simulink model "namestanje_parametara"  (R2018a)
settings: Solver=VariableStepAuto  StartTime=0.0  StopTime=10.0  RelTol=1e-3
values from neighbouring files (symbols this model uses):
  A = [ 0   1   0   0   0   0   0 ... (first row only)    [HPS.m]
  a21 = -4*k/(3*Mt)    (= -53333.3333333)    [HPS.m]
  a22 = -(Bp+b)/Mt    (= -13)    [HPS.m]
  a23 = Ap/Mt    (= 0.00065)    [HPS.m]
  a24 = 4*k/(3*Mt)    (= 53333.3333333)    [HPS.m]
  a25 = b/Mt    (= 10)    [HPS.m]
  a32 = -4*Be*Ap/Vt    (= -8450000000)    [HPS.m]
  a33 = -4*Be*(Ctp+Kc)/Vt    (= -2.6)    [HPS.m]
  a51 = 4*k/(3*m)    (= 26666.6666667)    [HPS.m]
  a52 = b/m    (= 5)    [HPS.m]
  a54 = -10*k/(3*m)    (= -66666.6666667)    [HPS.m]
  a55 = -(b+mu)/m    (= -5.001)    [HPS.m]
  a56 = 2*k/m    (= 40000)    [HPS.m]
  a74 = 4*k/m    (= 80000)    [HPS.m]
  a76 = -6*k/m    (= -120000)    [HPS.m]
  a77 = -2*mu/m    (= -0.002)    [HPS.m]
  Ap = D*D*pi/4    (= 0.00384845100065)    [HPS.m]
  B = [0;0;b31;0;0;0;0]    [HPS.m]
  b31 = 4*Be*Kq*Kt/(R*r*Kf*Vt)    (= 401440000)    [HPS.m]
  Bp = 30    [HPS.m]
  C = [0,0,0,1,0,0,0]    [HPS.m]
  DD = Kp*Td    (= 0.3675)    [HPS.m]
  I = Kp/Ti    (= 4800)    [HPS.m]
  Kp = 0.6*Kkr    (= 84)    [HPS.m]
  Mt = 10    [HPS.m]
libraries: simulink x2
settings Model: Creator=test4  LastModifiedBy=test4

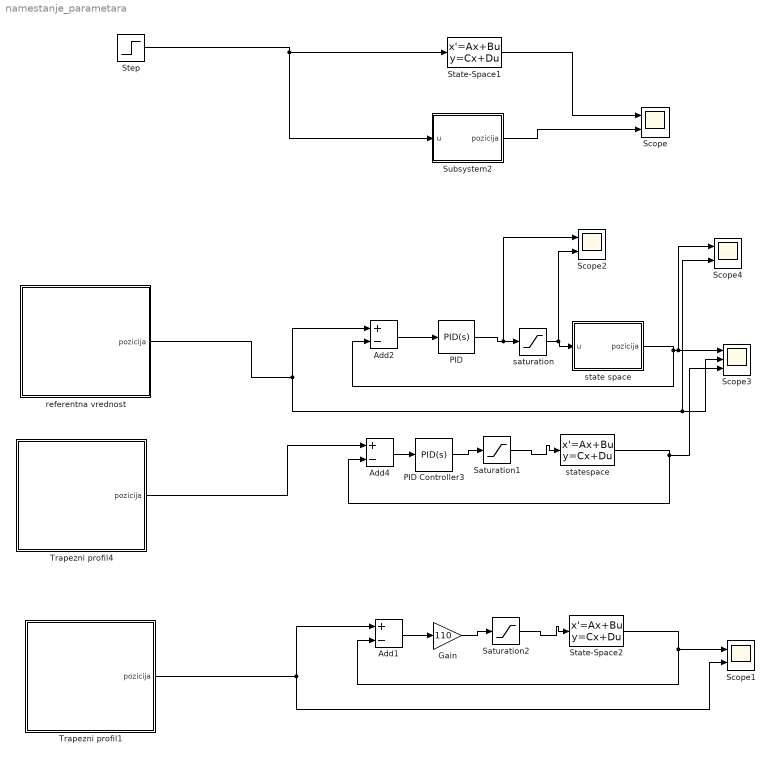
== system namestanje_parametara ==
  " PID" : simulink/Continuous/PID Controller  Controller=PID  TimeDomain=Continuous-time  SampleTime=-1  IntegratorMethod=Forward Euler  FilterMethod=Forward Euler  Form=Parallel  UseFilter=on  ControllerParametersSource=internal  P=Kp  I=I  D=DD  N=100  InitialConditionSource=internal  InitialConditionForIntegrator=0  InitialConditionForFilter=0  ExternalReset=none  LimitOutput=off  UpperSaturationLimit=inf  LowerSaturationLimit=-inf  LinearizeAsGain=on  AntiWindupMode=none  Kb=1  TrackingMode=off  Kt=1  PParamMin=[]  PParamMax=[]  IParamMin=[]  IParamMax=[]  DParamMin=[]  DParamMax=[]  NParamMin=[]  NParamMax=[]  KbParamMin=[]  KbParamMax=[]  KtParamMin=[]  KtParamMax=[]  POutMin=[]  POutMax=[]  IOutMin=[]  IOutMax=[]  DOutMin=[]  DOutMax=[]  NOutMin=[]  NOutMax=[]  KbOutMin=[]  KbOutMax=[]  KtOutMin=[]  KtOutMax=[]  IntegratorOutMin=[]  IntegratorOutMax=[]  FilterOutMin=[]  FilterOutMax=[]  SumOutMin=[]  SumOutMax=[]  SumI1OutMin=[]  SumI1OutMax=[]  SumI2OutMin=[]  SumI2OutMax=[]  SumI3OutMin=[]  SumI3OutMax=[]  SumDOutMin=[]  SumDOutMax=[]  SaturationOutMin=[]  SaturationOutMax=[]  IntegratorContinuousStateAttributes=''  IntegratorStateMustResolveToSignalObject=off  IntegratorRTWStateStorageClass=Auto  FilterContinuousStateAttributes=''  FilterStateMustResolveToSignalObject=off  FilterRTWStateStorageClass=Auto  DifferentiatorICPrevScaledInput=0  DifferentiatorOutMin=[]  DifferentiatorOutMax=[]  FilterDiffOutCoefMin=[]  FilterDiffOutCoefMax=[]  SumDenOutMin=[]  SumDenOutMax=[]  SumNumOutMin=[]  SumNumOutMax=[]  ReciprocalOutMin=[]  ReciprocalOutMax=[]  DivideOutMin=[]  DivideOutMax=[]  TunerSelectOption=Transfer Function Based (PID Tuner App)
  Add1 : Sum  Inputs=+-
  Add2 : Sum  Inputs=+-
  Add4 : Sum  Inputs=+-
  Gain : Gain  Gain=110
  PID Controller3 : simulink/Continuous/PID Controller  Controller=PID  TimeDomain=Continuous-time  SampleTime=-1  IntegratorMethod=Forward Euler  FilterMethod=Forward Euler  Form=Parallel  UseFilter=on  ControllerParametersSource=internal  P=Kp  I=I  D=DD  N=100  InitialConditionSource=internal  InitialConditionForIntegrator=0  InitialConditionForFilter=0  ExternalReset=none  LimitOutput=off  UpperSaturationLimit=inf  LowerSaturationLimit=-inf  LinearizeAsGain=on  AntiWindupMode=none  Kb=1  TrackingMode=off  Kt=1  PParamMin=[]  PParamMax=[]  IParamMin=[]  IParamMax=[]  DParamMin=[]  DParamMax=[]  NParamMin=[]  NParamMax=[]  KbParamMin=[]  KbParamMax=[]  KtParamMin=[]  KtParamMax=[]  POutMin=[]  POutMax=[]  IOutMin=[]  IOutMax=[]  DOutMin=[]  DOutMax=[]  NOutMin=[]  NOutMax=[]  KbOutMin=[]  KbOutMax=[]  KtOutMin=[]  KtOutMax=[]  IntegratorOutMin=[]  IntegratorOutMax=[]  FilterOutMin=[]  FilterOutMax=[]  SumOutMin=[]  SumOutMax=[]  SumI1OutMin=[]  SumI1OutMax=[]  SumI2OutMin=[]  SumI2OutMax=[]  SumI3OutMin=[]  SumI3OutMax=[]  SumDOutMin=[]  SumDOutMax=[]  SaturationOutMin=[]  SaturationOutMax=[]  IntegratorContinuousStateAttributes=''  IntegratorStateMustResolveToSignalObject=off  IntegratorRTWStateStorageClass=Auto  FilterContinuousStateAttributes=''  FilterStateMustResolveToSignalObject=off  FilterRTWStateStorageClass=Auto  DifferentiatorICPrevScaledInput=0  DifferentiatorOutMin=[]  DifferentiatorOutMax=[]  FilterDiffOutCoefMin=[]  FilterDiffOutCoefMax=[]  SumDenOutMin=[]  SumDenOutMax=[]  SumNumOutMin=[]  SumNumOutMax=[]  ReciprocalOutMin=[]  ReciprocalOutMax=[]  DivideOutMin=[]  DivideOutMax=[]  TunerSelectOption=Transfer Function Based (PID Tuner App)
  Saturation1 : Saturate  UpperLimit=24  LowerLimit=-24
  Saturation2 : Saturate  UpperLimit=24  LowerLimit=-24
  Scope{,1..2,4} (4 alike) : Scope  NumInputPorts=2
  Scope3 : Scope  NumInputPorts=3
  State-Space1 : StateSpace  A=A  B=B  C=C  D=0  InitialCondition=0
  State-Space2 : StateSpace  A=A  B=B  C=C  D=0  InitialCondition=0
  Step : Step  SampleTime=0
  Subsystem2 : Subsystem
  Trapezni profil1 : Subsystem
  Trapezni profil4 : Subsystem
  referentna vrednost : Subsystem
  saturation : Saturate  UpperLimit=24  LowerLimit=-24
  state space : Subsystem
  statespace : StateSpace  A=A  B=B  C=C  D=0  InitialCondition=0
  wires:
  State-Space1/1 -> Scope/1
  Subsystem2/1(pozicija) -> Scope/2
  Step/1 -> State-Space1/1, Subsystem2/1(u)
  " PID"/1 -> Scope2/1, saturation/1
  Trapezni profil1/1(pozicija) -> Scope1/2, Add1/1
  PID Controller3/1 -> Saturation1/1
  saturation/1 -> Scope2/2, state space/1(u)
  Gain/1 -> Saturation2/1
  Add2/1 -> " PID"/1
  Saturation1/1 -> statespace/1
  statespace/1 -> Scope3/3, Add4/2
  Add1/1 -> Gain/1
  Trapezni profil4/1(pozicija) -> Add4/1
  state space/1(pozicija) -> Scope4/1, Scope3/1, Add2/2
  referentna vrednost/1(pozicija) -> Add2/1, Scope4/2, Scope3/2
  Add4/1 -> PID Controller3/1
  State-Space2/1 -> Scope1/1, Add1/2
  Saturation2/1 -> State-Space2/1

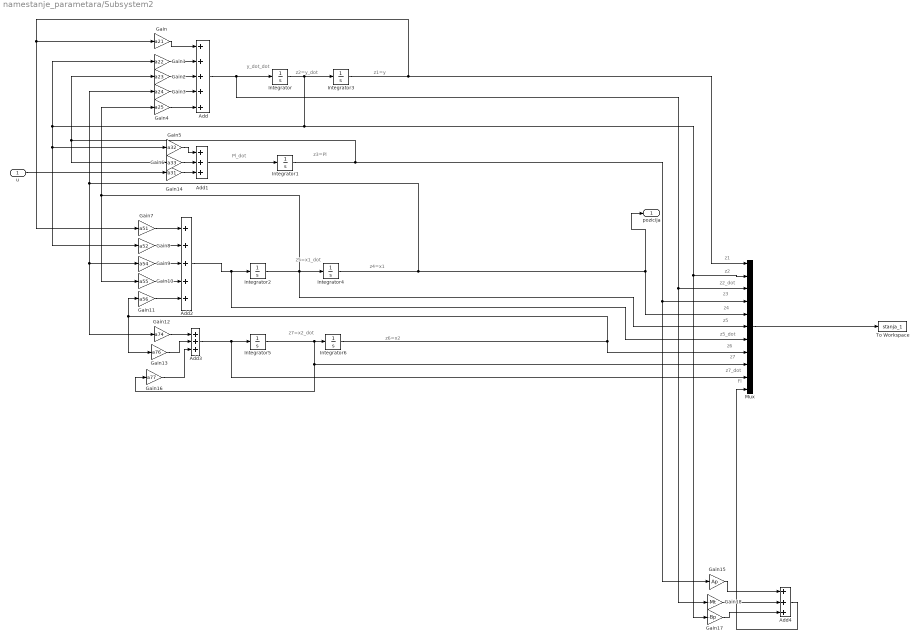
== system namestanje_parametara/Subsystem2 ==
  note: z3
  note: Fl
  note: z7_dot
  note: z7
  note: z6
  note: z5
  note: z4
  note: z2_dot
  note: z2
  note: z1
  note: z7=x2_dot
  note: z6=x2
  note: Pl_dot
  note: z5=x1_dot
  note: z4=x1
  note: y_dot_dot
  note: z3=Pl
  note: z1=y
  note: z2=y_dot
  note: z5_dot
  u : Inport
  Add : Sum  Inputs=+++++
  Add1 : Sum  Inputs=+++
  Add2 : Sum  Inputs=+++++
  Add3 : Sum  Inputs=+++
  Add4 : Sum  Inputs=+++
  Gain : Gain  Gain=a21
  Gain1 : Gain  Gain=a22
  Gain10 : Gain  Gain=a55
  Gain11 : Gain  Gain=a56
  Gain12 : Gain  Gain=a74
  Gain13 : Gain  Gain=a76
  Gain14 : Gain  Gain=b31
  Gain15 : Gain  Gain=Ap
  Gain16 : Gain  Gain=a77
  Gain17 : Gain  Gain=-Bp
  Gain18 : Gain  Gain=-Mt
  Gain2 : Gain  Gain=a23
  Gain3 : Gain  Gain=a24
  Gain4 : Gain  Gain=a25
  Gain5 : Gain  Gain=a32
  Gain6 : Gain  Gain=a33
  Gain7 : Gain  Gain=a51
  Gain8 : Gain  Gain=a52
  Gain9 : Gain  Gain=a54
  Integrator{,1..6} (7 alike) : Integrator
  Mux : Mux  Inputs=11
  To Workspace : ToWorkspace  VariableName=stanja_1  SampleTime=-1
  pozicija : Outport
  wires:
  Integrator/1 -> Mux/2, Gain17/1, Gain5/1, Gain8/1, Gain1/1, Integrator3/1
  Integrator4/1 -> Gain9/1, Gain12/1, Gain3/1, pozicija/1, Mux/5
  Gain13/1 -> Add3/2
  Gain4/1 -> Add/5
  Integrator5/1 -> Gain16/1, Mux/9, Integrator6/1
  Gain1/1 -> Add/2
  Add2/1 -> Mux/7, Integrator2/1
  Gain8/1 -> Add2/2
  Integrator6/1 -> Mux/8, Gain13/1, Gain11/1
  Add/1 -> Gain18/1, Mux/3, Integrator/1
  Gain6/1 -> Add1/2
  Gain2/1 -> Add/3
  Integrator1/1 -> Gain15/1, Mux/4, Gain6/1, Gain2/1
  Gain/1 -> Add/1
  Gain7/1 -> Add2/1
  Add3/1 -> Mux/10, Integrator5/1
  Gain10/1 -> Add2/4
  Add1/1 -> Integrator1/1
  Integrator3/1 -> Mux/1, Gain7/1, Gain/1
  Gain12/1 -> Add3/1
  Gain5/1 -> Add1/1
  Gain11/1 -> Add2/5
  Gain3/1 -> Add/4
  Gain9/1 -> Add2/3
  Integrator2/1 -> Mux/6, Integrator4/1, Gain4/1, Gain10/1
  Gain14/1 -> Add1/3
  u/1 -> Gain14/1
  Mux/1 -> To Workspace/1
  Gain18/1 -> Add4/2
  Gain15/1 -> Add4/1
  Gain17/1 -> Add4/3
  Add4/1 -> Mux/11
  Gain16/1 -> Add3/3

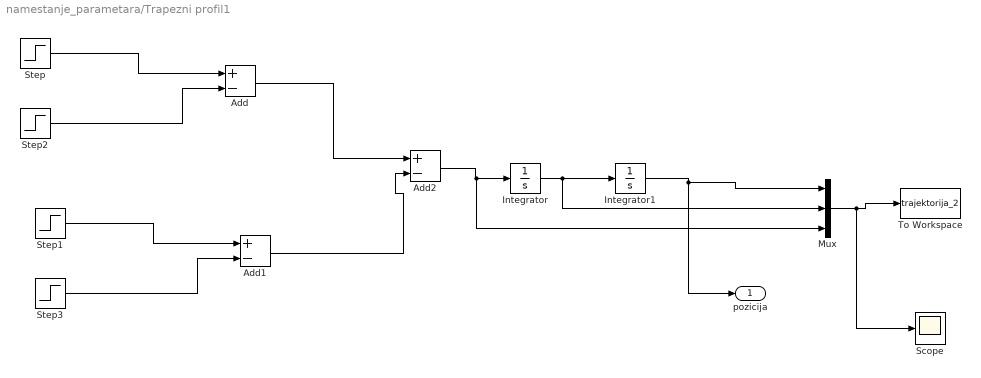
== system namestanje_parametara/Trapezni profil1 ==
  Add : Sum  Inputs=+-
  Add1 : Sum  Inputs=+-
  Add2 : Sum  Inputs=+-
  Integrator : Integrator
  Integrator1 : Integrator
  Mux : Mux  Inputs=3
  Scope : Scope
  Step : Step  Time=0  After=0.2667  SampleTime=0
  Step1 : Step  Time=1.5  After=0.2667  SampleTime=0
  Step2 : Step  Time=0.5  After=0.2667  SampleTime=0
  Step3 : Step  Time=2  After=0.2667  SampleTime=0
  To Workspace : ToWorkspace  VariableName=trajektorija_2  SampleTime=-1
  pozicija : Outport
  wires:
  Add1/1 -> Add2/2
  Step3/1 -> Add1/2
  Add/1 -> Add2/1
  Integrator1/1 -> Mux/1, pozicija/1
  Integrator/1 -> Mux/2, Integrator1/1
  Add2/1 -> Mux/3, Integrator/1
  Step1/1 -> Add1/1
  Step2/1 -> Add/2
  Step/1 -> Add/1
  Mux/1 -> Scope/1, To Workspace/1

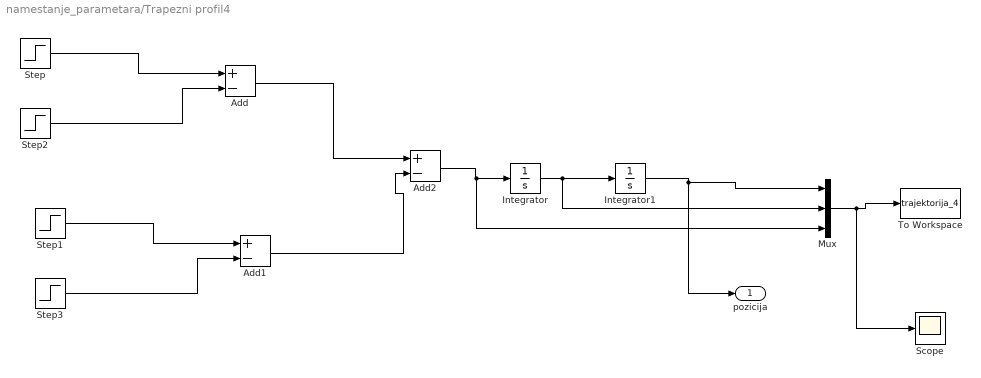
== system namestanje_parametara/Trapezni profil4 ==
  Add : Sum  Inputs=+-
  Add1 : Sum  Inputs=+-
  Add2 : Sum  Inputs=+-
  Integrator : Integrator
  Integrator1 : Integrator
  Mux : Mux  Inputs=3
  Scope : Scope
  Step : Step  Time=0  After=0.2667  SampleTime=0
  Step1 : Step  Time=1.5  After=0.2667  SampleTime=0
  Step2 : Step  Time=0.5  After=0.2667  SampleTime=0
  Step3 : Step  Time=2  After=0.2667  SampleTime=0
  To Workspace : ToWorkspace  VariableName=trajektorija_4  SampleTime=-1
  pozicija : Outport
  wires:
  Add1/1 -> Add2/2
  Step3/1 -> Add1/2
  Add/1 -> Add2/1
  Integrator1/1 -> Mux/1, pozicija/1
  Integrator/1 -> Mux/2, Integrator1/1
  Add2/1 -> Mux/3, Integrator/1
  Step1/1 -> Add1/1
  Step2/1 -> Add/2
  Step/1 -> Add/1
  Mux/1 -> Scope/1, To Workspace/1

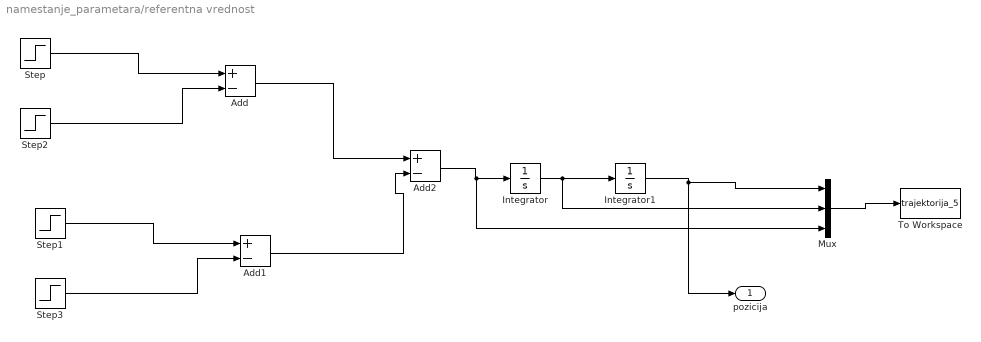
== system namestanje_parametara/referentna vrednost ==
  Add : Sum  Inputs=+-
  Add1 : Sum  Inputs=+-
  Add2 : Sum  Inputs=+-
  Integrator : Integrator
  Integrator1 : Integrator
  Mux : Mux  Inputs=3
  Step : Step  Time=0  After=0.2667  SampleTime=0
  Step1 : Step  Time=1.5  After=0.2667  SampleTime=0
  Step2 : Step  Time=0.5  After=0.2667  SampleTime=0
  Step3 : Step  Time=2  After=0.2667  SampleTime=0
  To Workspace : ToWorkspace  VariableName=trajektorija_5  SampleTime=-1
  pozicija : Outport
  wires:
  Add1/1 -> Add2/2
  Step3/1 -> Add1/2
  Add/1 -> Add2/1
  Integrator1/1 -> Mux/1, pozicija/1
  Integrator/1 -> Mux/2, Integrator1/1
  Add2/1 -> Mux/3, Integrator/1
  Step1/1 -> Add1/1
  Step2/1 -> Add/2
  Step/1 -> Add/1
  Mux/1 -> To Workspace/1

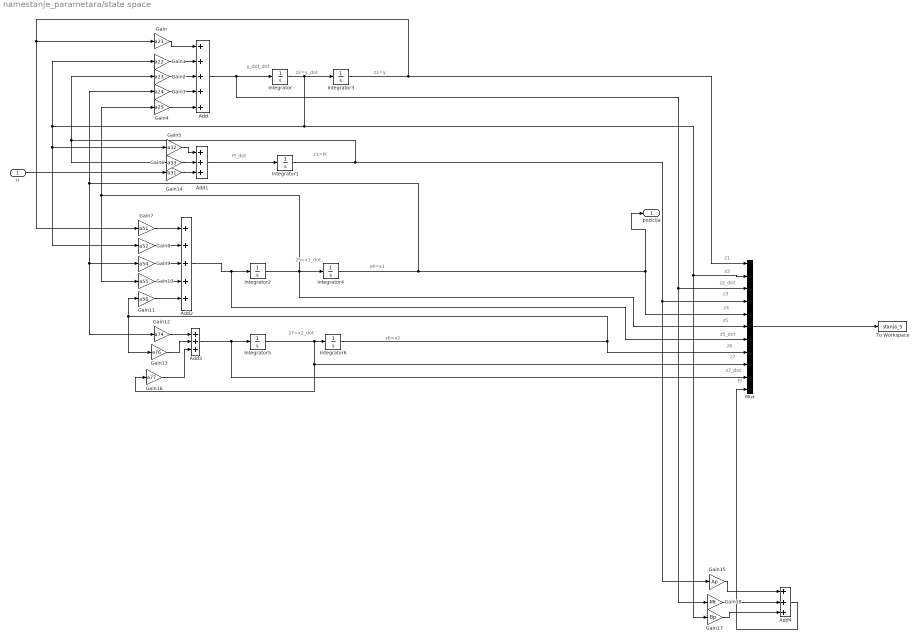
== system namestanje_parametara/state space ==
  note: z3
  note: Fl
  note: z7_dot
  note: z7
  note: z6
  note: z5
  note: z4
  note: z2_dot
  note: z2
  note: z1
  note: z7=x2_dot
  note: z6=x2
  note: Pl_dot
  note: z5=x1_dot
  note: z4=x1
  note: y_dot_dot
  note: z3=Pl
  note: z1=y
  note: z2=y_dot
  note: z5_dot
  u : Inport
  Add : Sum  Inputs=+++++
  Add1 : Sum  Inputs=+++
  Add2 : Sum  Inputs=+++++
  Add3 : Sum  Inputs=+++
  Add4 : Sum  Inputs=+++
  Gain : Gain  Gain=a21
  Gain1 : Gain  Gain=a22
  Gain10 : Gain  Gain=a55
  Gain11 : Gain  Gain=a56
  Gain12 : Gain  Gain=a74
  Gain13 : Gain  Gain=a76
  Gain14 : Gain  Gain=b31
  Gain15 : Gain  Gain=Ap
  Gain16 : Gain  Gain=a77
  Gain17 : Gain  Gain=-Bp
  Gain18 : Gain  Gain=-Mt
  Gain2 : Gain  Gain=a23
  Gain3 : Gain  Gain=a24
  Gain4 : Gain  Gain=a25
  Gain5 : Gain  Gain=a32
  Gain6 : Gain  Gain=a33
  Gain7 : Gain  Gain=a51
  Gain8 : Gain  Gain=a52
  Gain9 : Gain  Gain=a54
  Integrator{,1..6} (7 alike) : Integrator
  Mux : Mux  Inputs=11
  To Workspace : ToWorkspace  VariableName=stanja_5  SampleTime=-1
  pozicija : Outport
  wires:
  Integrator/1 -> Mux/2, Gain17/1, Gain5/1, Gain8/1, Gain1/1, Integrator3/1
  Integrator4/1 -> Gain9/1, Gain12/1, Gain3/1, pozicija/1, Mux/5
  Gain13/1 -> Add3/2
  Gain4/1 -> Add/5
  Integrator5/1 -> Gain16/1, Mux/9, Integrator6/1
  Gain1/1 -> Add/2
  Add2/1 -> Mux/7, Integrator2/1
  Gain8/1 -> Add2/2
  Integrator6/1 -> Mux/8, Gain13/1, Gain11/1
  Add/1 -> Gain18/1, Mux/3, Integrator/1
  Gain6/1 -> Add1/2
  Gain2/1 -> Add/3
  Integrator1/1 -> Gain15/1, Mux/4, Gain6/1, Gain2/1
  Gain/1 -> Add/1
  Gain7/1 -> Add2/1
  Add3/1 -> Mux/10, Integrator5/1
  Gain10/1 -> Add2/4
  Add1/1 -> Integrator1/1
  Integrator3/1 -> Mux/1, Gain7/1, Gain/1
  Gain12/1 -> Add3/1
  Gain5/1 -> Add1/1
  Gain11/1 -> Add2/5
  Gain3/1 -> Add/4
  Gain9/1 -> Add2/3
  Integrator2/1 -> Mux/6, Integrator4/1, Gain4/1, Gain10/1
  Gain14/1 -> Add1/3
  u/1 -> Gain14/1
  Mux/1 -> To Workspace/1
  Gain18/1 -> Add4/2
  Gain15/1 -> Add4/1
  Gain17/1 -> Add4/3
  Add4/1 -> Mux/11
  Gain16/1 -> Add3/3
